simulink model "CL_Xpro_model"  (Simulink 9.0)
settings: Solver=ode45  StartTime=0.0  StopTime=100  RelTol=1e-3  EnableMultiTasking=on
values from neighbouring files (symbols this model uses):
  a1 = 16.235    [LoadQuadrotorConst_XPro1a.m]
  a2 = 17.912    [LoadQuadrotorConst_XPro1a.m]
  a3 = 17.914    [LoadQuadrotorConst_XPro1a.m]
  a4 = 18.161    [LoadQuadrotorConst_XPro1a.m]
  b1 = -0.5036    [LoadQuadrotorConst_XPro1a.m]
  b2 = -12.728    [LoadQuadrotorConst_XPro1a.m]
  b3 = -6.5646    [LoadQuadrotorConst_XPro1a.m]
  b4 = -7.4637    [LoadQuadrotorConst_XPro1a.m]
  c = 0.0002    [LoadQuadrotorConst_XPro1a.m]
  c_mi_x = 170    [LoadQuadrotorConst_XPro1a.m]
  c_mi_y = 170    [LoadQuadrotorConst_XPro1a.m]
  c_mi_z = 40    [LoadQuadrotorConst_XPro1a.m]
  co_x = 1.7    [LoadQuadrotorConst_XPro1a.m]
  co_y = 1.7    [LoadQuadrotorConst_XPro1a.m]
  co_z = 90.7    [LoadQuadrotorConst_XPro1a.m]
  d = 0.0071    [LoadQuadrotorConst_XPro1a.m]
  d_omega_R10 = 9.1275    [initial_conditions.m]
  d_omega_R20 = 8.955    [initial_conditions.m]
  d_omega_R30 = 8.61    [initial_conditions.m]
  d_omega_R40 = 8.543    [initial_conditions.m]
  dfi_0 = 0    [initial_conditions.m]
  dpsi_0 = 0    [initial_conditions.m]
  dtheta_0 = 0    [initial_conditions.m]
  dx_0 = 0    [initial_conditions.m]
  dy_0 = 0    [initial_conditions.m]
  dz_0 = 0    [initial_conditions.m]
  f = 5e-6    (= 5e-06)    [LoadQuadrotorConst_XPro1a.m]
  fi_0 = 0    [initial_conditions.m]
  g = 0.0008    [LoadQuadrotorConst_XPro1a.m]    (also in cvx_guidance.m = [0; 0; -9.81])
  ga = 9.807    [LoadQuadrotorConst_XPro1a.m]
  h = -0.0282    [LoadQuadrotorConst_XPro1a.m]
  hover = [V1_WP;V2_WP;V3_WP;V4_WP]    [initial_conditions.m]
  Ixx = 2.1385*100    (= 213.85)    [LoadQuadrotorConst_XPro1a.m]
  Iyy = Ixx    (= 213.85)    [LoadQuadrotorConst_XPro1a.m]
  Izz = 3.7479*100    (= 374.79)    [LoadQuadrotorConst_XPro1a.m]
  Jr = 4.86851*0.1    (= 0.486851)    [LoadQuadrotorConst_XPro1a.m]
  K = C(1:4,:)    [newthingtest2.m]
  L = 0.422    [LoadQuadrotorConst_XPro1a.m]
  m = 2.1    [LoadQuadrotorConst_XPro1a.m]    (also in cvx_guidance.m; plot_all_data3D.m = exp(z))
  psi_0 = 0    [initial_conditions.m]
  Tau = 0.1    [LoadQuadrotorConst_XPro1a.m]
  theta_0 = 0    [initial_conditions.m]
  V1_WP = 9.1275    [initial_conditions.m]
  V2_WP = 8.955    [initial_conditions.m]
  V3_WP = 8.61    [initial_conditions.m]
  V4_WP = 8.543    [initial_conditions.m]
  x_0 = 0    [initial_conditions.m]
  y_0 = 0    [initial_conditions.m]
  z_0 = 30    [initial_conditions.m]
undefined symbols (not defined in the file or in its folder): bb, dd, Xref
settings Model: Creator=Jake  LastModifiedBy=Padraig Lysandrou
settings DataIOCC: LimitDataPoints=on  SignalLoggingSaveFormat=ModelDataLogs
settings OptimizationCC: InitFltsAndDblsToZero=on
settings DebuggingCC: SaveWithParameterizedLinksMsg=none  SignalResolutionControl=TryResolveAllWithWarning  SolverPrmCheckMsg=warning  MultiTaskDSMMsg=warning  MultiTaskCondExecSysMsg=none  FcnCallInpInsideContextMsg=warning  StrictBusMsg=Warning
settings SFSimCC: SimParseCustomCode=off
settings GRTTargetCC: TargetFcnLib=ansi_tfl_tmw.mat  CombineOutputUpdateFcns=off  GRTInterface=on

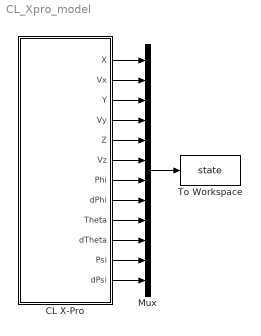
== system CL_Xpro_model ==
  CL X-Pro : Subsystem
  Mux : Mux  Inputs=12
  To Workspace : ToWorkspace  VariableName=state  SaveFormat=Timeseries  SampleTime=-1
  wires:
  Mux/1 -> To Workspace/1
  CL X-Pro/1(X) -> Mux/1
  CL X-Pro/2(Vx) -> Mux/2
  CL X-Pro/3(Y) -> Mux/3
  CL X-Pro/4(Vy) -> Mux/4
  CL X-Pro/5(Z) -> Mux/5
  CL X-Pro/6(Vz) -> Mux/6
  CL X-Pro/7(Phi) -> Mux/7
  CL X-Pro/8(dPhi) -> Mux/8
  CL X-Pro/9(Theta) -> Mux/9
  CL X-Pro/10(dTheta) -> Mux/10
  CL X-Pro/11(Psi) -> Mux/11
  CL X-Pro/12(dPsi) -> Mux/12

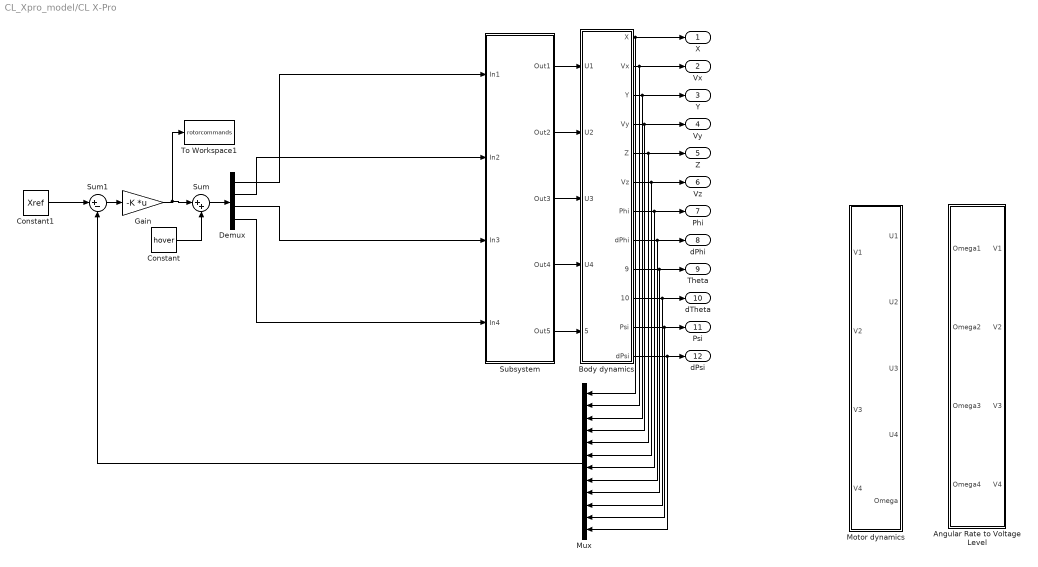
== system CL_Xpro_model/CL X-Pro ==
  Angular Rate to Voltage Level : Subsystem
  Body dynamics : Subsystem
  Constant : Constant  Value=hover
  Constant1 : Constant  Value=Xref
  Demux : Demux
  Gain : Gain  Gain=-K  Multiplication=Matrix(K*u) (u vector)
  Motor dynamics : Subsystem
  Mux : Mux  Inputs=12
  Subsystem : Subsystem
  Sum : Sum  Inputs=|++
  Sum1 : Sum  Inputs=|+-
  To Workspace1 : ToWorkspace  VariableName=rotorcommands  SaveFormat=Timeseries  SampleTime=-1
  X : Outport
  Vx : Outport  Port=2
  Y : Outport  Port=3
  Vy : Outport  Port=4
  Z : Outport  Port=5
  Vz : Outport  Port=6
  Phi : Outport  Port=7
  dPhi : Outport  Port=8
  Theta : Outport  Port=9
  dTheta : Outport  Port=10
  Psi : Outport  Port=11
  dPsi : Outport  Port=12
  wires:
  Body dynamics/1(X) -> Mux/1, X/1
  Body dynamics/2("Vx ") -> Mux/2, Vx/1
  Body dynamics/3(Y) -> Y/1, Mux/3
  Body dynamics/4(Vy) -> Mux/4, Vy/1
  Body dynamics/5(Z) -> Mux/5, Z/1
  Body dynamics/6("Vz ") -> Mux/6, Vz/1
  Body dynamics/7(Phi) -> Mux/7, Phi/1
  Body dynamics/11(Psi) -> Mux/11, Psi/1
  Body dynamics/9(Theta) -> Mux/9, Theta/1
  Body dynamics/8(dPhi) -> Mux/8, dPhi/1
  Body dynamics/10(dTheta) -> Mux/10, dTheta/1
  Body dynamics/12(dPsi) -> Mux/12, dPsi/1
  Constant1/1 -> Sum1/1
  Mux/1 -> Sum1/2
  Sum1/1 -> Gain/1
  Gain/1 -> Sum/1, To Workspace1/1
  Subsystem/5(Out5) -> Body dynamics/5(Omega)
  Subsystem/4(Out4) -> Body dynamics/4(U4)
  Subsystem/3(Out3) -> Body dynamics/3(U3)
  Subsystem/2(Out2) -> Body dynamics/2(U2)
  Subsystem/1(Out1) -> Body dynamics/1(U1)
  Demux/1 -> Subsystem/1(In1)
  Demux/2 -> Subsystem/2(In2)
  Demux/3 -> Subsystem/3(In3)
  Demux/4 -> Subsystem/4(In4)
  Sum/1 -> Demux/1
  Constant/1 -> Sum/2

== system CL_Xpro_model/CL X-Pro/Angular Rate to Voltage Level ==
  Omega1 : Inport
  Omega2 : Inport  Port=2
  Omega3 : Inport  Port=3
  Omega4 : Inport  Port=4
  reverseR1 : Subsystem
  reverseR2 : Subsystem
  reverseR3 : Subsystem
  reverseR4 : Subsystem
  V1 : Outport
  V2 : Outport  Port=2
  V3 : Outport  Port=3
  V4 : Outport  Port=4
  wires:
  reverseR3/1(V1) -> V3/1
  Omega2/1 -> reverseR2/1(Omega)
  reverseR4/1(V1) -> V4/1
  reverseR1/1(V1) -> V1/1
  Omega3/1 -> reverseR3/1(Omega)
  Omega4/1 -> reverseR4/1(Omega)
  reverseR2/1(V1) -> V2/1
  Omega1/1 -> reverseR1/1(Omega)

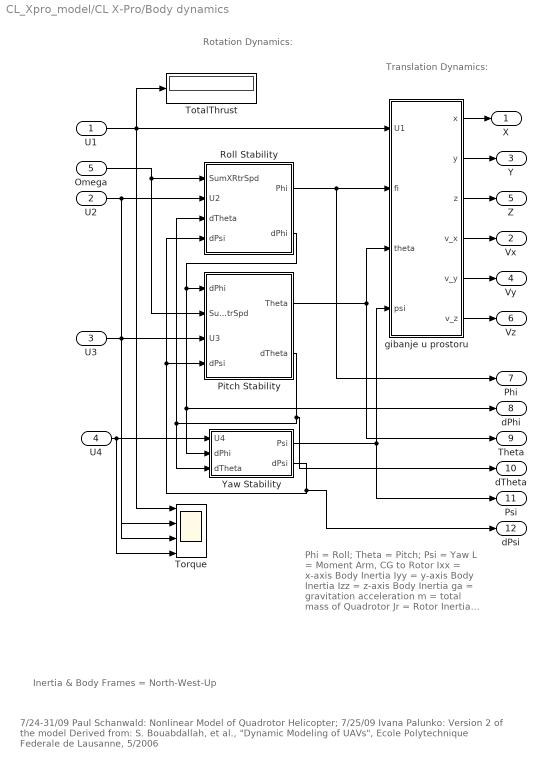
== system CL_Xpro_model/CL X-Pro/Body dynamics ==
  note: Inertia & Body Frames = North-West-Up
  note: Rotation
      | Dynamics:
  note: Translation
      | Dynamics:
  note: Phi = Roll; Theta = Pitch; Psi = Yaw
      | L = Moment Arm, CG to Rotor
      | Ixx = x-axis Body Inertia
      | Iyy = y-axis Body Inertia
      | Izz = z-axis Body Inertia
      | ga = gravitation acceleration
      | m = total mass of Quadrotor
      | Jr = Rotor Inertia
      | a,b = Volts-to-Rotor Speed Consts
      | c,d,e = RtrSpd-to-Thrust Fcn Consts
      | f,g,h = RtrSpd-to-Drag Fcn Consts
      | Tau = Motor Time Const
  note: 7/24-31/09  Paul Schanwald:  Nonlinear Model of Quadrotor Helicopter; 7/25/09 Ivana Palunko: Version 2 of the model
      | Derived from: S. Bouabdallah, et al., "Dynamic Modeling of UAVs", Ecole Polytechnique Federale de Lausanne, 5/2006
  U1 : Inport
  U2 : Inport  Port=2
  U3 : Inport  Port=3
  U4 : Inport  Port=4
  Omega : Inport  Port=5
  Pitch Stability : Subsystem
  Roll Stability : Subsystem
  Torque : Scope  NumInputPorts=4
  TotalThrust : Display
  Yaw Stability : Subsystem
  gibanje u prostoru : Subsystem
  X : Outport
  "Vx " : Outport  Port=2
  Y : Outport  Port=3
  Vy : Outport  Port=4
  Z : Outport  Port=5
  "Vz " : Outport  Port=6
  Phi : Outport  Port=7
  dPhi : Outport  Port=8
  Theta : Outport  Port=9
  dTheta : Outport  Port=10
  Psi : Outport  Port=11
  dPsi : Outport  Port=12
  wires:
  U4/1 -> Yaw Stability/1(U4), Torque/4
  U3/1 -> Pitch Stability/3(U3), Torque/3
  U1/1 -> TotalThrust/1, gibanje u prostoru/1(U1), Torque/1
  gibanje u prostoru/3(z) -> Z/1
  gibanje u prostoru/2(y) -> Y/1
  gibanje u prostoru/1(x) -> X/1
  U2/1 -> Roll Stability/2(U2), Torque/2
  Omega/1 -> Roll Stability/1(SumXRtrSpd), Pitch Stability/2(SumYRtrSpd)
  Roll Stability/2(dPhi) -> Pitch Stability/1(dPhi), dPhi/1, Yaw Stability/2(dPhi)
  Pitch Stability/2(dTheta) -> dTheta/1, Yaw Stability/3(dTheta), Roll Stability/3(dTheta)
  Yaw Stability/2(dPsi) -> dPsi/1, Roll Stability/4(dPsi), Pitch Stability/4(dPsi)
  Roll Stability/1(Phi) -> gibanje u prostoru/2(fi), Phi/1
  Pitch Stability/1(Theta) -> gibanje u prostoru/3(theta), Theta/1
  Yaw Stability/1(Psi) -> Psi/1, gibanje u prostoru/4(psi)
  gibanje u prostoru/6(v_z) -> "Vz "/1
  gibanje u prostoru/4(v_x) -> "Vx "/1
  gibanje u prostoru/5(v_y) -> Vy/1

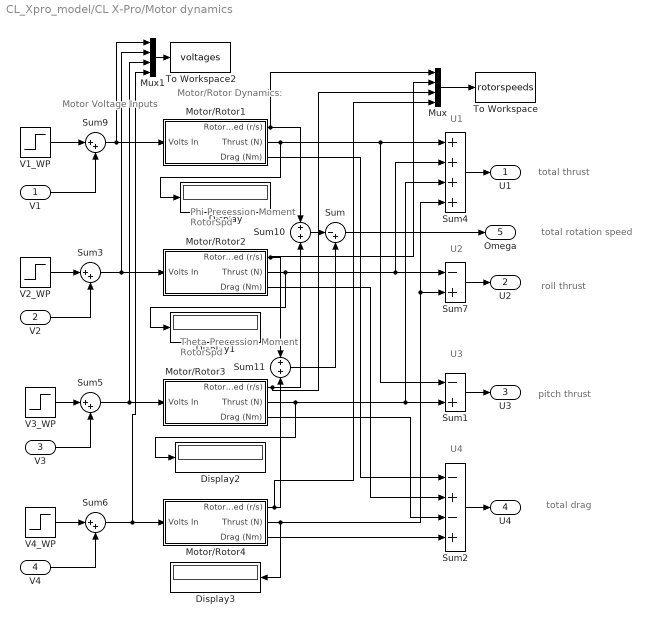
== system CL_Xpro_model/CL X-Pro/Motor dynamics ==
  note: total drag
  note: pitch thrust
  note: roll thrust
  note: total rotation speed
  note: total thrust
  note: Theta Precession
      | Moment RotorSpd
  note: Phi Precession
      | Moment RotorSpd
  note: Motor/Rotor
      | Dynamics:
  note: Motor
      | Voltage
      | Inputs
  note: U4
  note: U3
  note: U2
  note: U1
  V1 : Inport
  V2 : Inport  Port=2
  V3 : Inport  Port=3
  V4 : Inport  Port=4
  Display{,1..3} (4 alike) : Display
  Motor/Rotor1 : Subsystem
  Motor/Rotor2 : Subsystem
  Motor/Rotor3 : Subsystem
  Motor/Rotor4 : Subsystem
  Mux : Mux
  Mux1 : Mux
  Sum : Sum  Inputs=|-+
  Sum1 : Sum  Inputs=-+
  Sum10 : Sum  Inputs=+|+
  Sum11 : Sum  Inputs=+|+
  Sum2 : Sum  Inputs=-+-+
  Sum{3,5..6,9} (4 alike) : Sum  Inputs=|++
  Sum4 : Sum  Inputs=++++
  Sum7 : Sum  Inputs=-+
  To Workspace : ToWorkspace  VariableName=rotorspeeds  SaveFormat=Timeseries  SampleTime=-1
  To Workspace2 : ToWorkspace  VariableName=voltages  SaveFormat=Timeseries  SampleTime=-1
  V1_WP : Step  Time=0  Before=V1_WP  After=V1_WP  SampleTime=0
  V2_WP : Step  Time=0  Before=V2_WP  After=V2_WP  SampleTime=0
  V3_WP : Step  Time=0  Before=V3_WP  After=V3_WP  SampleTime=0
  V4_WP : Step  Time=0  Before=V4_WP  After=V4_WP  SampleTime=0
  U1 : Outport
  U2 : Outport  Port=2
  U3 : Outport  Port=3
  U4 : Outport  Port=4
  Omega : Outport  Port=5
  wires:
  Sum11/1 -> Sum/2
  Sum10/1 -> Sum/1
  Motor/Rotor4/1(Rotor Speed (r/s)) -> Mux/4, Sum11/2
  Motor/Rotor4/2(Thrust (N)) -> Display3/1, Sum4/4, Sum7/2
  Motor/Rotor4/3(Drag (Nm)) -> Sum2/4
  Motor/Rotor3/3(Drag (Nm)) -> Sum2/3
  Motor/Rotor3/1(Rotor Speed (r/s)) -> Mux/3, Sum10/2
  Motor/Rotor3/2(Thrust (N)) -> Display2/1, Sum4/3, Sum1/2
  Motor/Rotor2/1(Rotor Speed (r/s)) -> Mux/2, Sum11/1
  Motor/Rotor2/3(Drag (Nm)) -> Sum2/2
  Motor/Rotor2/2(Thrust (N)) -> Display1/1, Sum4/2, Sum7/1
  Motor/Rotor1/1(Rotor Speed (r/s)) -> Mux/1, Sum10/1
  Motor/Rotor1/3(Drag (Nm)) -> Sum2/1
  Motor/Rotor1/2(Thrust (N)) -> Display/1, Sum4/1, Sum1/1
  Sum4/1 -> U1/1
  Sum/1 -> Omega/1
  Sum7/1 -> U2/1
  Sum1/1 -> U3/1
  Sum2/1 -> U4/1
  Sum9/1 -> Mux1/1, Motor/Rotor1/1(Volts In)
  V1_WP/1 -> Sum9/1
  V2_WP/1 -> Sum3/1
  Sum3/1 -> Mux1/2, Motor/Rotor2/1(Volts In)
  V3_WP/1 -> Sum5/1
  Sum5/1 -> Mux1/3, Motor/Rotor3/1(Volts In)
  V4_WP/1 -> Sum6/1
  Sum6/1 -> Mux1/4, Motor/Rotor4/1(Volts In)
  V1/1 -> Sum9/2
  V2/1 -> Sum3/2
  V3/1 -> Sum5/2
  V4/1 -> Sum6/2
  Mux/1 -> To Workspace/1
  Mux1/1 -> To Workspace2/1

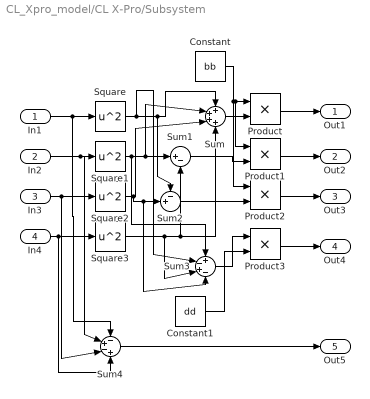
== system CL_Xpro_model/CL X-Pro/Subsystem ==
  In1 : Inport
  In2 : Inport  Port=2
  In3 : Inport  Port=3
  In4 : Inport  Port=4
  Constant : Constant  Value=bb
  Constant1 : Constant  Value=dd
  Product{,1..3} (4 alike) : Product
  Square{,1..3} (4 alike) : Math  Operator=square  RndMeth=Zero  SaturateOnIntegerOverflow=on
  Sum : Sum  Inputs=4
  Sum1 : Sum  Inputs=|+-
  Sum2 : Sum  Inputs=-+|
  Sum3 : Sum  Inputs=+-+-
  Sum4 : Sum  Inputs=-+-+
  Out1 : Outport
  Out2 : Outport  Port=2
  Out3 : Outport  Port=3
  Out4 : Outport  Port=4
  Out5 : Outport  Port=5
  wires:
  In1/1 -> Sum4/1, Square/1
  In2/1 -> Sum4/2, Square1/1
  In3/1 -> Sum4/3, Square2/1
  In4/1 -> Sum4/4, Square3/1
  Square/1 -> Sum3/2, Sum2/1, Sum/1
  Square1/1 -> Sum3/1, Sum1/1, Sum/2
  Square2/1 -> Sum3/4, Sum2/2, Sum/3
  Square3/1 -> Sum3/3, Sum1/2, Sum/4
  Sum/1 -> Product/2
  Constant/1 -> Product1/1, Product/1, Product2/1
  Product/1 -> Out1/1
  Product1/1 -> Out2/1
  Sum1/1 -> Product1/2
  Sum2/1 -> Product2/2
  Product2/1 -> Out3/1
  Product3/1 -> Out4/1
  Sum3/1 -> Product3/1
  Constant1/1 -> Product3/2
  Sum4/1 -> Out5/1

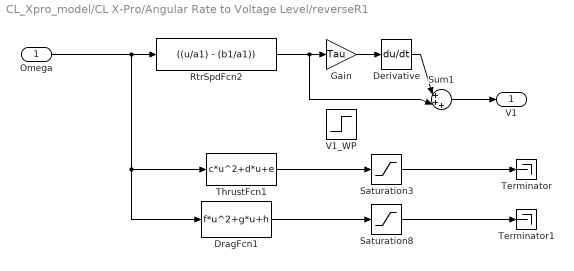
== system CL_Xpro_model/CL X-Pro/Angular Rate to Voltage Level/reverseR1 ==
  Omega : Inport
  Derivative : Derivative
  DragFcn1 : Fcn  Expr=f*u^2+g*u+h
  Gain : Gain  Gain=Tau
  RtrSpdFcn2 : Fcn  Expr=((u/a1) - (b1/a1))
  Saturation3 : Saturate  UpperLimit=15  LowerLimit=0
  Saturation8 : Saturate  UpperLimit=1  LowerLimit=0
  Sum1 : Sum  Inputs=|+++
  Terminator : Terminator
  Terminator1 : Terminator
  ThrustFcn1 : Fcn  Expr=c*u^2+d*u+e
  V1_WP : Step  Time=0  Before=V1_WP  After=V1_WP  SampleTime=0
  V1 : Outport
  wires:
  Derivative/1 -> Sum1/1
  RtrSpdFcn2/1 -> Sum1/2, Gain/1
  Sum1/1 -> V1/1
  Omega/1 -> RtrSpdFcn2/1, ThrustFcn1/1, DragFcn1/1
  DragFcn1/1 -> Saturation8/1
  Saturation8/1 -> Terminator1/1
  ThrustFcn1/1 -> Saturation3/1
  Saturation3/1 -> Terminator/1
  Gain/1 -> Derivative/1

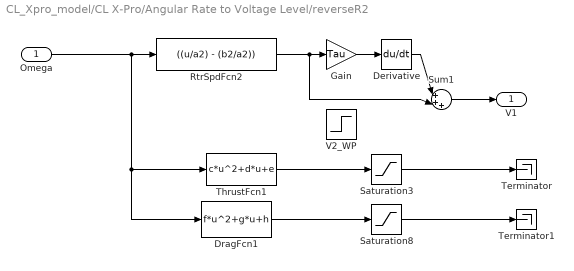
== system CL_Xpro_model/CL X-Pro/Angular Rate to Voltage Level/reverseR2 ==
  Omega : Inport
  Derivative : Derivative
  DragFcn1 : Fcn  Expr=f*u^2+g*u+h
  Gain : Gain  Gain=Tau
  RtrSpdFcn2 : Fcn  Expr=((u/a2) - (b2/a2))
  Saturation3 : Saturate  UpperLimit=15  LowerLimit=0
  Saturation8 : Saturate  UpperLimit=1  LowerLimit=0
  Sum1 : Sum  Inputs=|+++
  Terminator : Terminator
  Terminator1 : Terminator
  ThrustFcn1 : Fcn  Expr=c*u^2+d*u+e
  V2_WP : Step  Time=0  Before=V2_WP  After=V2_WP  SampleTime=0
  V1 : Outport
  wires:
  Derivative/1 -> Sum1/1
  RtrSpdFcn2/1 -> Sum1/2, Gain/1
  Sum1/1 -> V1/1
  Omega/1 -> RtrSpdFcn2/1, ThrustFcn1/1, DragFcn1/1
  DragFcn1/1 -> Saturation8/1
  Saturation8/1 -> Terminator1/1
  ThrustFcn1/1 -> Saturation3/1
  Saturation3/1 -> Terminator/1
  Gain/1 -> Derivative/1

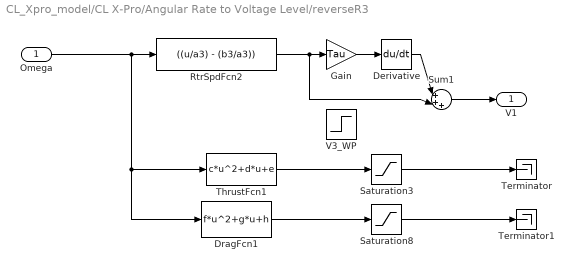
== system CL_Xpro_model/CL X-Pro/Angular Rate to Voltage Level/reverseR3 ==
  Omega : Inport
  Derivative : Derivative
  DragFcn1 : Fcn  Expr=f*u^2+g*u+h
  Gain : Gain  Gain=Tau
  RtrSpdFcn2 : Fcn  Expr=((u/a3) - (b3/a3))
  Saturation3 : Saturate  UpperLimit=15  LowerLimit=0
  Saturation8 : Saturate  UpperLimit=1  LowerLimit=0
  Sum1 : Sum  Inputs=|+++
  Terminator : Terminator
  Terminator1 : Terminator
  ThrustFcn1 : Fcn  Expr=c*u^2+d*u+e
  V3_WP : Step  Time=0  Before=V3_WP  After=V3_WP  SampleTime=0
  V1 : Outport
  wires:
  Derivative/1 -> Sum1/1
  RtrSpdFcn2/1 -> Sum1/2, Gain/1
  Sum1/1 -> V1/1
  Omega/1 -> RtrSpdFcn2/1, ThrustFcn1/1, DragFcn1/1
  DragFcn1/1 -> Saturation8/1
  Saturation8/1 -> Terminator1/1
  ThrustFcn1/1 -> Saturation3/1
  Saturation3/1 -> Terminator/1
  Gain/1 -> Derivative/1

== system CL_Xpro_model/CL X-Pro/Angular Rate to Voltage Level/reverseR4 ==
  Omega : Inport
  Derivative : Derivative
  DragFcn1 : Fcn  Expr=f*u^2+g*u+h
  Gain : Gain  Gain=Tau
  RtrSpdFcn2 : Fcn  Expr=((u/a4) - (b4/a4))
  Saturation3 : Saturate  UpperLimit=15  LowerLimit=0
  Saturation8 : Saturate  UpperLimit=1  LowerLimit=0
  Sum1 : Sum  Inputs=|+++
  Terminator : Terminator
  Terminator1 : Terminator
  ThrustFcn1 : Fcn  Expr=c*u^2+d*u+e
  V4_WP : Step  Time=0  Before=V4_WP  After=V4_WP  SampleTime=0
  V1 : Outport
  wires:
  Derivative/1 -> Sum1/1
  RtrSpdFcn2/1 -> Sum1/2, Gain/1
  Sum1/1 -> V1/1
  Omega/1 -> RtrSpdFcn2/1, ThrustFcn1/1, DragFcn1/1
  DragFcn1/1 -> Saturation8/1
  Saturation8/1 -> Terminator1/1
  ThrustFcn1/1 -> Saturation3/1
  Saturation3/1 -> Terminator/1
  Gain/1 -> Derivative/1

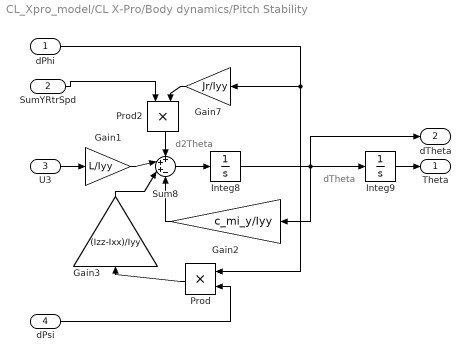
== system CL_Xpro_model/CL X-Pro/Body dynamics/Pitch Stability ==
  note: d2Theta
  note: dTheta
  dPhi : Inport
  SumYRtrSpd : Inport  Port=2
  U3 : Inport  Port=3
  dPsi : Inport  Port=4
  Gain1 : Gain  Gain=L/Iyy
  Gain2 : Gain  Gain=c_mi_y/Iyy
  Gain3 : Gain  Gain=(Izz-Ixx)/Iyy
  Gain7 : Gain  Gain=Jr/Iyy
  Integ8 : Integrator  InitialCondition=dtheta_0
  Integ9 : Integrator  InitialCondition=theta_0  UpperSaturationLimit=pi/2  LowerSaturationLimit=-pi/2
  Prod : Product  RndMeth=Zero
  Prod2 : Product  RndMeth=Zero
  Sum8 : Sum  Inputs=+++-
  Theta : Outport
  dTheta : Outport  Port=2
  wires:
  Gain2/1 -> Sum8/4
  dPhi/1 -> Prod/1, Gain7/1
  Integ9/1 -> Theta/1
  U3/1 -> Gain1/1
  SumYRtrSpd/1 -> Prod2/1
  dPsi/1 -> Prod/2
  Integ8/1 -> dTheta/1, Integ9/1, Gain2/1
  Sum8/1 -> Integ8/1
  Gain1/1 -> Sum8/2
  Gain7/1 -> Prod2/2
  Gain3/1 -> Sum8/3
  Prod/1 -> Gain3/1
  Prod2/1 -> Sum8/1

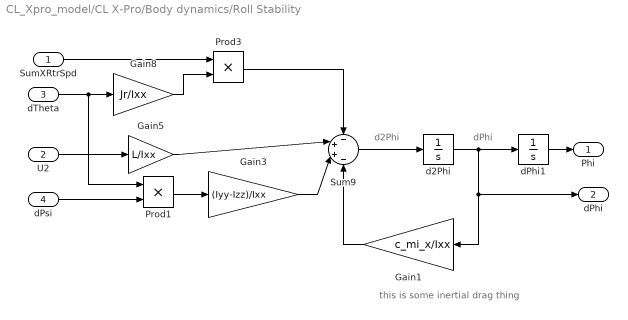
== system CL_Xpro_model/CL X-Pro/Body dynamics/Roll Stability ==
  note: this is some inertial drag thing
  note: d2Phi
  note: dPhi
  SumXRtrSpd : Inport
  U2 : Inport  Port=2
  dTheta : Inport  Port=3
  dPsi : Inport  Port=4
  Gain1 : Gain  Gain=c_mi_x/Ixx
  Gain3 : Gain  Gain=(Iyy-Izz)/Ixx
  Gain5 : Gain  Gain=L/Ixx
  Gain8 : Gain  Gain=Jr/Ixx
  Prod1 : Product  RndMeth=Zero
  Prod3 : Product  RndMeth=Zero
  Sum9 : Sum  Inputs=-++-
  d2Phi : Integrator  InitialCondition=dfi_0
  dPhi1 : Integrator  InitialCondition=fi_0  UpperSaturationLimit=pi/2  LowerSaturationLimit=-pi/2
  Phi : Outport
  dPhi : Outport  Port=2
  wires:
  dPsi/1 -> Prod1/2
  dTheta/1 -> Prod1/1, Gain8/1
  Prod3/1 -> Sum9/1
  SumXRtrSpd/1 -> Prod3/1
  Gain8/1 -> Prod3/2
  dPhi1/1 -> Phi/1
  U2/1 -> Gain5/1
  d2Phi/1 -> Gain1/1, dPhi/1, dPhi1/1
  Sum9/1 -> d2Phi/1
  Gain5/1 -> Sum9/2
  Gain1/1 -> Sum9/4
  Gain3/1 -> Sum9/3
  Prod1/1 -> Gain3/1

== system CL_Xpro_model/CL X-Pro/Body dynamics/Yaw Stability ==
  note: dPsi
  note: d2Psi
  U4 : Inport
  dPhi : Inport  Port=2
  dTheta : Inport  Port=3
  Gain : Gain  Gain=1/Izz
  Gain1 : Gain  Gain=c_mi_z
  Gain2 : Gain  Gain=Ixx-Iyy
  Integ10 : Integrator  InitialCondition=dpsi_0
  Integ11 : Integrator  InitialCondition=psi_0
  Product : Product  RndMeth=Zero
  Sum : Sum  Inputs=|++-
  Psi : Outport
  dPsi : Outport  Port=2
  wires:
  Sum/1 -> Gain/1
  U4/1 -> Sum/1
  Integ11/1 -> Psi/1
  Gain/1 -> Integ10/1
  Integ10/1 -> Gain1/1, dPsi/1, Integ11/1
  Gain1/1 -> Sum/3
  Gain2/1 -> Sum/2
  dPhi/1 -> Product/1
  dTheta/1 -> Product/2
  Product/1 -> Gain2/1

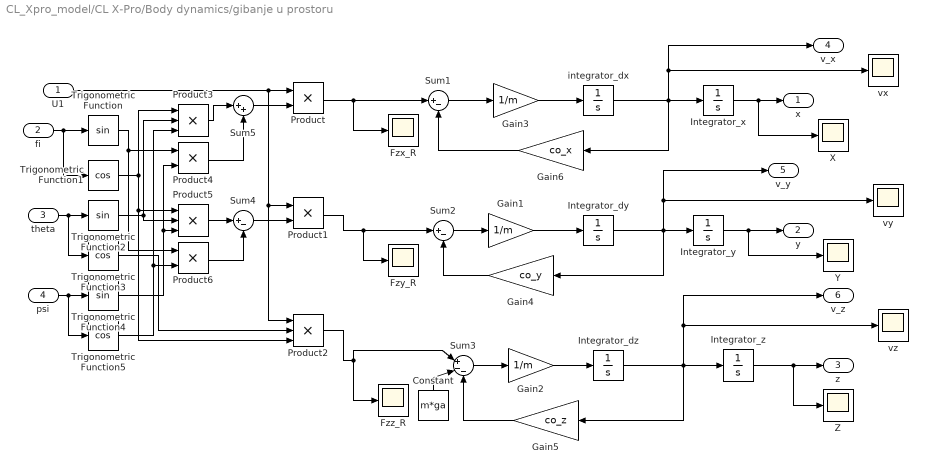
== system CL_Xpro_model/CL X-Pro/Body dynamics/gibanje u prostoru ==
  U1 : Inport
  fi : Inport  Port=2
  theta : Inport  Port=3
  psi : Inport  Port=4
  Constant : Constant  Value=m*ga
  Fzx_R : Scope
  Fzy_R : Scope
  Fzz_R : Scope
  Gain1 : Gain  Gain=1/m
  Gain2 : Gain  Gain=1/m
  Gain3 : Gain  Gain=1/m
  Gain4 : Gain  Gain=co_y
  Gain5 : Gain  Gain=co_z
  Gain6 : Gain  Gain=co_x
  Integrator_dy : Integrator  InitialCondition=dy_0  LimitOutput=on  UpperSaturationLimit=10  LowerSaturationLimit=-10
  Integrator_dz : Integrator  InitialCondition=dz_0  LimitOutput=on  UpperSaturationLimit=10  LowerSaturationLimit=-10
  Integrator_x : Integrator  InitialCondition=x_0
  Integrator_y : Integrator  InitialCondition=y_0
  Integrator_z : Integrator  InitialCondition=z_0
  Product{,1,4,6} (4 alike) : Product  RndMeth=Zero
  Product2 : Product  Inputs=3  RndMeth=Zero
  Product3 : Product  Inputs=3  RndMeth=Zero
  Product5 : Product  Inputs=3  RndMeth=Zero
  Sum1 : Sum  Inputs=|+-
  Sum2 : Sum  Inputs=|+-
  Sum3 : Sum  Inputs=|+--
  Sum4 : Sum  Inputs=|+-
  Sum5 : Sum  Inputs=|++
  Trigonometric Function : Trigonometry
  Trigonometric Function1 : Trigonometry  Operator=cos
  Trigonometric Function2 : Trigonometry
  Trigonometric Function3 : Trigonometry  Operator=cos
  Trigonometric Function4 : Trigonometry
  Trigonometric Function5 : Trigonometry  Operator=cos
  X : Scope
  Y : Scope
  Z : Scope
  integrator_dx : Integrator  InitialCondition=dx_0  LimitOutput=on  UpperSaturationLimit=10  LowerSaturationLimit=-10
  vx : Scope
  vy : Scope
  vz : Scope
  x : Outport
  y : Outport  Port=2
  z : Outport  Port=3
  v_x : Outport  Port=4
  v_y : Outport  Port=5
  v_z : Outport  Port=6
  wires:
  Gain5/1 -> Sum3/3
  Constant/1 -> Sum3/2
  Gain4/1 -> Sum2/2
  Sum3/1 -> Gain2/1
  Gain6/1 -> Sum1/2
  Product2/1 -> Sum3/1, Fzz_R/1
  Sum2/1 -> Gain1/1
  Product1/1 -> Fzy_R/1, Sum2/1
  Gain2/1 -> Integrator_dz/1
  Sum1/1 -> Gain3/1
  Product/1 -> Fzx_R/1, Sum1/1
  U1/1 -> Product/1, Product1/1, Product2/1
  Integrator_y/1 -> Y/1, y/1
  Integrator_x/1 -> X/1, x/1
  Integrator_z/1 -> Z/1, z/1
  integrator_dx/1 -> Gain6/1, vx/1, v_x/1, Integrator_x/1
  Integrator_dy/1 -> Gain4/1, Integrator_y/1, vy/1, v_y/1
  Integrator_dz/1 -> vz/1, v_z/1, Gain5/1, Integrator_z/1
  Gain1/1 -> Integrator_dy/1
  Gain3/1 -> integrator_dx/1
  Sum4/1 -> Product1/2
  Sum5/1 -> Product/2
  Product3/1 -> Sum5/1
  Product4/1 -> Sum5/2
  Product5/1 -> Sum4/1
  Product6/1 -> Sum4/2
  psi/1 -> Trigonometric Function4/1, Trigonometric Function5/1
  theta/1 -> Trigonometric Function2/1, Trigonometric Function3/1
  fi/1 -> Trigonometric Function/1, Trigonometric Function1/1
  Trigonometric Function/1 -> Product4/1, Product6/1
  Trigonometric Function1/1 -> Product3/1, Product5/1, Product2/3
  Trigonometric Function2/1 -> Product3/2, Product5/2
  Trigonometric Function5/1 -> Product3/3, Product6/2
  Trigonometric Function4/1 -> Product4/2, Product5/3
  Trigonometric Function3/1 -> Product2/2

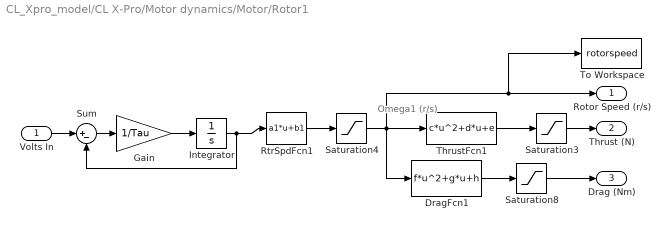
== system CL_Xpro_model/CL X-Pro/Motor dynamics/Motor/Rotor1 ==
  note: Omega1
      | (r/s)
  Volts In : Inport
  DragFcn1 : Fcn  Expr=f*u^2+g*u+h
  Gain : Gain  Gain=1/Tau
  Integrator : Integrator  InitialCondition=d_omega_R10
  RtrSpdFcn1 : Fcn  Expr=a1*u+b1
  Saturation3 : Saturate  UpperLimit=15  LowerLimit=0
  Saturation4 : Saturate  UpperLimit=250  LowerLimit=0
  Saturation8 : Saturate  UpperLimit=1  LowerLimit=0
  Sum : Sum  Inputs=|+-
  ThrustFcn1 : Fcn  Expr=c*u^2+d*u+e
  To Workspace : ToWorkspace  VariableName=rotorspeed  SaveFormat=Timeseries  SampleTime=-1
  Rotor Speed (r/s) : Outport
  Thrust (N) : Outport  Port=2
  Drag (Nm) : Outport  Port=3
  wires:
  Volts In/1 -> Sum/1
  Sum/1 -> Gain/1
  Integrator/1 -> RtrSpdFcn1/1, Sum/2
  Gain/1 -> Integrator/1
  Saturation3/1 -> Thrust (N)/1
  Saturation8/1 -> Drag (Nm)/1
  DragFcn1/1 -> Saturation8/1
  Saturation4/1 -> To Workspace/1, Rotor Speed (r/s)/1, DragFcn1/1, ThrustFcn1/1
  RtrSpdFcn1/1 -> Saturation4/1
  ThrustFcn1/1 -> Saturation3/1

== system CL_Xpro_model/CL X-Pro/Motor dynamics/Motor/Rotor2 ==
  note: Omega1
      | (r/s)
  Volts In : Inport
  DragFcn1 : Fcn  Expr=f*u^2+g*u+h
  Gain : Gain  Gain=1/Tau
  Integrator : Integrator  InitialCondition=d_omega_R20
  RtrSpdFcn1 : Fcn  Expr=a2*u+b2
  Saturation3 : Saturate  UpperLimit=15  LowerLimit=0
  Saturation4 : Saturate  UpperLimit=250  LowerLimit=0
  Saturation8 : Saturate  UpperLimit=1  LowerLimit=0
  Sum : Sum  Inputs=|+-
  ThrustFcn1 : Fcn  Expr=c*u^2+d*u+e
  Rotor Speed (r/s) : Outport
  Thrust (N) : Outport  Port=2
  Drag (Nm) : Outport  Port=3
  wires:
  Volts In/1 -> Sum/1
  Sum/1 -> Gain/1
  Integrator/1 -> RtrSpdFcn1/1, Sum/2
  Gain/1 -> Integrator/1
  Saturation3/1 -> Thrust (N)/1
  Saturation8/1 -> Drag (Nm)/1
  DragFcn1/1 -> Saturation8/1
  ThrustFcn1/1 -> Saturation3/1
  Saturation4/1 -> Rotor Speed (r/s)/1, DragFcn1/1, ThrustFcn1/1
  RtrSpdFcn1/1 -> Saturation4/1

== system CL_Xpro_model/CL X-Pro/Motor dynamics/Motor/Rotor3 ==
  note: Omega1
      | (r/s)
  Volts In : Inport
  DragFcn1 : Fcn  Expr=f*u^2+g*u+h
  Gain : Gain  Gain=1/Tau
  Integrator : Integrator  InitialCondition=d_omega_R30
  RtrSpdFcn1 : Fcn  Expr=a3*u+b3
  Saturation3 : Saturate  UpperLimit=15  LowerLimit=0
  Saturation4 : Saturate  UpperLimit=250  LowerLimit=0
  Saturation8 : Saturate  UpperLimit=1  LowerLimit=0
  Sum : Sum  Inputs=|+-
  ThrustFcn1 : Fcn  Expr=c*u^2+d*u+e
  Rotor Speed (r/s) : Outport
  Thrust (N) : Outport  Port=2
  Drag (Nm) : Outport  Port=3
  wires:
  Volts In/1 -> Sum/1
  Sum/1 -> Gain/1
  Integrator/1 -> RtrSpdFcn1/1, Sum/2
  Gain/1 -> Integrator/1
  Saturation3/1 -> Thrust (N)/1
  Saturation8/1 -> Drag (Nm)/1
  DragFcn1/1 -> Saturation8/1
  ThrustFcn1/1 -> Saturation3/1
  Saturation4/1 -> Rotor Speed (r/s)/1, DragFcn1/1, ThrustFcn1/1
  RtrSpdFcn1/1 -> Saturation4/1

== system CL_Xpro_model/CL X-Pro/Motor dynamics/Motor/Rotor4 ==
  note: Omega1
      | (r/s)
  Volts In : Inport
  DragFcn1 : Fcn  Expr=f*u^2+g*u+h
  Gain : Gain  Gain=1/Tau
  Integrator : Integrator  InitialCondition=d_omega_R40
  RtrSpdFcn1 : Fcn  Expr=a4*u+b4
  Saturation3 : Saturate  UpperLimit=15  LowerLimit=0
  Saturation4 : Saturate  UpperLimit=250  LowerLimit=0
  Saturation8 : Saturate  UpperLimit=1  LowerLimit=0
  Sum : Sum  Inputs=|+-
  ThrustFcn1 : Fcn  Expr=c*u^2+d*u+e
  Rotor Speed (r/s) : Outport
  Thrust (N) : Outport  Port=2
  Drag (Nm) : Outport  Port=3
  wires:
  Volts In/1 -> Sum/1
  Sum/1 -> Gain/1
  Integrator/1 -> RtrSpdFcn1/1, Sum/2
  Gain/1 -> Integrator/1
  Saturation3/1 -> Thrust (N)/1
  Saturation8/1 -> Drag (Nm)/1
  DragFcn1/1 -> Saturation8/1
  ThrustFcn1/1 -> Saturation3/1
  Saturation4/1 -> Rotor Speed (r/s)/1, DragFcn1/1, ThrustFcn1/1
  RtrSpdFcn1/1 -> Saturation4/1
